simulink model "OSWEC"  (R2025b)
settings: Solver=ode14x  StartTime=0  StopTime=400  FixedStep=0.01  MaxStep=0.01  RelTol=1e-3  EnableMultiTasking=on
values from neighbouring files (symbols this model uses):
  accVolHP = 50*0.5    (= 25)    [VariableDefinition.m]
  crankLength = 3    [VariableDefinition.m]
  Dmax = 42    [VariableDefinition.m]
  genShaftSpeedRef = 1800    [VariableDefinition.m]
  iGainGen = 1    [VariableDefinition.m]
  m3persecond2lpm = 1000*60    (= 60000)    [VariableDefinition.m]
  offsetLength = 1.3    [VariableDefinition.m]
  pa2psi = 1/6894.75    (= 0.000145037891149)    [VariableDefinition.m]
  pGainGen = 5    [VariableDefinition.m]
  radsec2rpm = 60/(2*pi)    (= 9.54929658551)    [VariableDefinition.m]
  rodLength = 5    [VariableDefinition.m]
undefined symbols (not defined in the file or in its folder): body, constraint, pto
libraries: fl_lib x55, nesl_utility x28, sh_lib x9, WECSim_Lib_Body_Elements x2, WECSim_Lib_Constraints x1, WECSim_Lib_Frames x1, WECSim_Lib_PTOs x1, slpidlib x1, sdl_lib x1
settings Model: Creator=mlawson  LastModifiedBy=jleonqu
settings SolverCC: ZeroCrossControl=DisableAll  AlgebraicLoopSolver=LineSearch  AutoInsertRateTranBlk=on
settings DataIOCC: SaveFormat=Array  SaveOutput=off  SaveTime=off  ReturnWorkspaceOutputs=off
settings OptimizationCC: LifeSpan=inf  SimCompilerOptimization=on
settings DebuggingCC: MergeDetectMultiDrivingBlocksExec=none  SolverPrmCheckMsg=warning  UnconnectedInputMsg=warning  UnconnectedOutputMsg=warning  UnconnectedLineMsg=warning  AllowSymbolicDim=off  StateNameClashWarn=warning  SFUnexpectedBacktrackingDiag=warning  SFNoUnconditionalDefaultTransitionDiag=warning  SFExecutionAtInitializationDiag=none  ArithmeticOperatorsInVariantConditions=warning
settings HardwareCC: ProdBitPerPointer=32.0  ProdBitPerSizeT=32.0  ProdBitPerPtrDiffT=32.0  ProdLargestAtomicFloat=None  ProdIntDivRoundTo=Undefined  ProdEndianess=Unspecified  ProdWordSize=32.0  ProdHWDeviceType=32-bit Generic
settings ModelReferenceCC: EnableRefExpFcnMdlSchedulingChecks=on  PropagateSignalLabelsOutOfModel=off
settings SFSimCC: SimUseLocalCustomCode=off  CustomCodeUndefinedFunction=UseInterfaceOnly
settings RTWCC: RTWUseLocalCustomCode=off  GPUComputeCapability=3.5  DLArmComputeVersion=19.05
settings CodeAppCC: StateflowObjectComments=on
settings GRTTargetCC: TargetLangStandard=C89/C90 (ANSI)
settings ConfigComp: CovMetricSettings=dw  CovSaveCumulativeToWorkspaceVar=on  CovSaveSingleToWorkspaceVar=on  CovExternalEMLEnable=off  CovSFcnEnable=off
settings SimscapeCC: SimscapeNormalizeSystem=off
settings ConfigurationSet: Description=SimMechanics 2G
settings ExplorerConfigSet: SimMechanicsOpenEditorOnUpdate=off  InternalSimMechanicsExplorerSettings="<ExplorerConfiguration><canonicalview>default</canonicalview><TilePanel><TileInfo><Tiles Columns=\"1\" Count=\"1\" Rows=\"1\"><Column Left=\"2\" Weight=\"1\"/><Column Left=\"1335\"/><Row Top=\"2\" Weight=\"1\"/><Row Top=\"911\"/><Tile Height=\"1\" Width=\"1\" X=\"0\" Y=\"0\"/></Tiles></TileInfo><SceneInfo><SceneViewer><BGColor><R>0.60000002384185791</R><G>0.60000002384185791</G><B>0.60000002384185791</B></BGColor><Camera><Position><X>365.37645888990272</X><Y>-369.82486814446582</Y><Z>359.64809521743916</Z></Position><Center><X>-6.7351450971904585</X><Y>2.2867358426280204</Y><Z>-12.463508769654169</Z></Center><Up><X>-0.40824829046386307</X><Y>0.40824829046386307</Y><Z>0.81649658092772615</Z></Up><Left>-57.820127362122818</Left><Right>57.820127362122818</Right><Bottom>-38.308817187253304</Bottom><Top>38.308817187253304</Top></Camera></SceneViewer></SceneInfo></TilePanel></ExplorerConfiguration>"

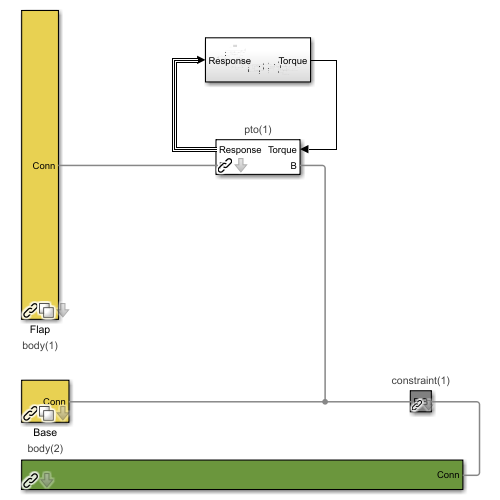
[thumbnail: Simulink's stored preview of the top-level diagram]
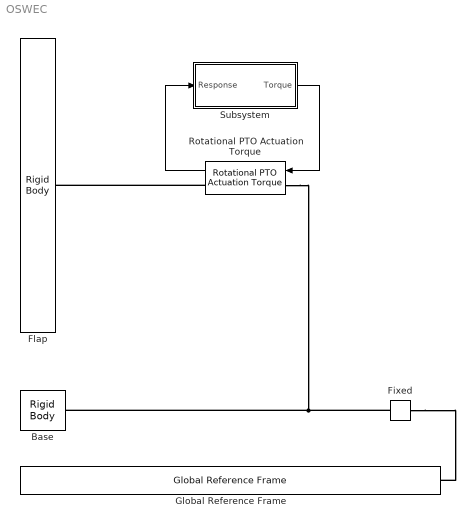
== system OSWEC ==
  Base : WECSim_Lib_Body_Elements/Rigid Body  body=body(2)
      settings: SourceProductName=WEC-Sim
  Fixed : WECSim_Lib_Constraints/Fixed  constraint=constraint(1)
      settings: AttributesFormatString=%<constraint>  SourceProductName=WEC-Sim
  Flap : WECSim_Lib_Body_Elements/Rigid Body  body=body(1)
      settings: SourceProductName=WEC-Sim
  Global Reference Frame : WECSim_Lib_Frames/Global Reference Frame  waves=waves  simu=simu
      settings: SourceProductName=WEC-Sim
  Rotational PTO Actuation Torque : WECSim_Lib_PTOs/Rotational PTO Actuation Torque  pto=pto(1)
      settings: AttributesFormatString=%<pto>
  Subsystem : Subsystem
  wires:
  Rotational PTO Actuation Torque/1 -> Subsystem/1(Response)
  Subsystem/1(Torque) -> Rotational PTO Actuation Torque/1
  connections:
  Fixed/LConn1 -- Global Reference Frame/RConn1
  Fixed/RConn1 -- Rotational PTO Actuation Torque/LConn1 -- Base/RConn1
  Rotational PTO Actuation Torque/RConn1 -- Flap/RConn1

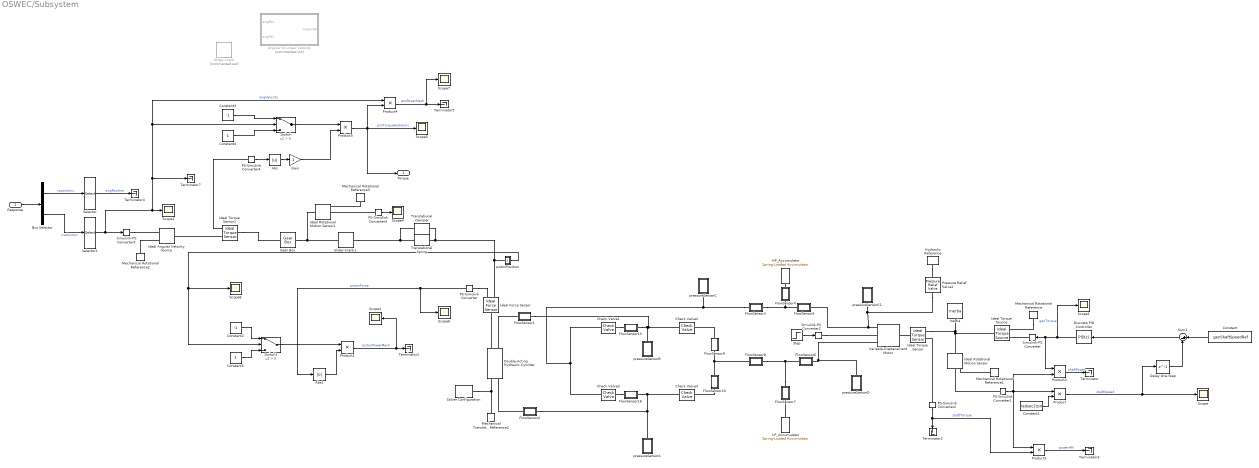
== system OSWEC/Subsystem ==
  Response : Inport
  Abs : Abs  SaturateOnIntegerOverflow=off
  Abs1 : Abs  SaturateOnIntegerOverflow=off
  Angular to Linear Velocity : Subsystem  Commented=on  AncestorBlock=|
      | WECSim_Lib_PTOSim/Motion Conversion/Rotary to Linear
      | Crank/Angular to Linear
      | Velocity
  Bus Selector : BusSelector  OutputSignals=position,velocity
  Check Valve1 : sh_lib/Valves/Directional Valves/Check Valve  area_max=areaMaxValve m^2  pres_crack=pCrack psi  pres_max=pMaxValve psi  C_d=0.7  A_leak=1e-12 m^2  lam_spec=1  B_lam=0.999  Re_cr=12  dynamic=0  tau=0.1 s  area_init=1e-12 m^2
      settings: InternalSimscapePortConfiguration="{\"Bottom\":[],\"Left\":[{\"id\":\"A\",\"label\":\"A\",\"type\":\"foundation.hydraulic.hydraulic\"}],\"Right\":[{\"id\":\"B\",\"label\":\"B\",\"type\":\"foundation.hydraulic.hydraulic\"}],\"Top\":[]}"
  Check Valve2 : sh_lib/Valves/Directional Valves/Check Valve  area_max=areaMaxValveLP m^2  pres_crack=pCrackLP psi  pres_max=pMaxValveLP psi  C_d=0.7  A_leak=1e-12 m^2  lam_spec=1  B_lam=0.999  Re_cr=12  dynamic=0  tau=0.1 s  area_init=1e-12 m^2
      settings: InternalSimscapePortConfiguration="{\"Bottom\":[],\"Left\":[{\"id\":\"A\",\"label\":\"A\",\"type\":\"foundation.hydraulic.hydraulic\"}],\"Right\":[{\"id\":\"B\",\"label\":\"B\",\"type\":\"foundation.hydraulic.hydraulic\"}],\"Top\":[]}"
  Check Valve3 : sh_lib/Valves/Directional Valves/Check Valve  area_max=areaMaxValve m^2  pres_crack=pCrack psi  pres_max=pMaxValve psi  C_d=0.7  A_leak=1e-12 m^2  lam_spec=1  B_lam=0.999  Re_cr=12  dynamic=0  tau=0.1 s  area_init=1e-12 m^2
      settings: InternalSimscapePortConfiguration="{\"Bottom\":[],\"Left\":[{\"id\":\"A\",\"label\":\"A\",\"type\":\"foundation.hydraulic.hydraulic\"}],\"Right\":[{\"id\":\"B\",\"label\":\"B\",\"type\":\"foundation.hydraulic.hydraulic\"}],\"Top\":[]}"
  Check Valve4 : sh_lib/Valves/Directional Valves/Check Valve  area_max=areaMaxValveLP m^2  pres_crack=pCrackLP psi  pres_max=pMaxValveLP psi  C_d=0.7  A_leak=1e-12 m^2  lam_spec=1  B_lam=0.999  Re_cr=12  dynamic=0  tau=0.1 s  area_init=1e-12 m^2
      settings: InternalSimscapePortConfiguration="{\"Bottom\":[],\"Left\":[{\"id\":\"A\",\"label\":\"A\",\"type\":\"foundation.hydraulic.hydraulic\"}],\"Right\":[{\"id\":\"B\",\"label\":\"B\",\"type\":\"foundation.hydraulic.hydraulic\"}],\"Top\":[]}"
  Constant : Constant  Value=genShaftSpeedRef
  Constant1 : Constant  Value=radsec2rpm
  Constant2 : Constant  Value=-1
  Constant3 : Constant  Value=-1
  Constant4 : Constant
  Constant5 : Constant
  Delay One Step : Delay  DelayLength=1
  Discrete PID Controller : slpidlib/PID Controller  Controller=PID  Form=Parallel  TimeDomain=Discrete-time  UseExternalTs=off  SampleTime=-1  IntegratorMethod=Forward Euler  FilterMethod=Forward Euler  ControllerParametersSource=internal  P=pGainGen  I=iGainGen  UseKiTs=off  D=0  UseExternalDerivativeSource=off  N=100  UseFilter=off  TunerSelectOption=Transfer Function Based (PID Tuner App)  InitialConditionSource=internal  InitialConditionForIntegrator=0  InitialConditionForFilter=0  DifferentiatorICPrevScaledInput=0  ExternalReset=none  TrackingMode=off  Kt=1  LimitOutput=off  SatLimitsSource=internal  UpperSaturationLimit=inf  LowerSaturationLimit=-inf  LinearizeAsGain=off  AntiWindupMode=none  Kb=1  LimitIntegrator=off  UpperIntegratorSaturationLimit=inf  LowerIntegratorSaturationLimit=-inf  POutMin=[]  POutMax=[]  IOutMin=[]  IOutMax=[]  DOutMin=[]  DOutMax=[]  NOutMin=[]  NOutMax=[]  SumOutMin=[]  SumOutMax=[]  SaturationOutMin=[]  SaturationOutMax=[]  PParamMin=[]  PParamMax=[]  IParamMin=[]  IParamMax=[]  DParamMin=[]  DParamMax=[]  NParamMin=[]  NParamMax=[]  KbParamMin=[]  KbParamMax=[]  KtParamMin=[]  KtParamMax=[]  KbOutMin=[]  KbOutMax=[]  KtOutMin=[]  KtOutMax=[]  IntegratorOutMin=[]  IntegratorOutMax=[]  FilterOutMin=[]  FilterOutMax=[]  SumI1OutMin=[]  SumI1OutMax=[]  SumI2OutMin=[]  SumI2OutMax=[]  SumI3OutMin=[]  SumI3OutMax=[]  SumI4OutMin=[]  SumI4OutMax=[]  SumDOutMin=[]  SumDOutMax=[]  DifferentiatorOutMin=[]  DifferentiatorOutMax=[]  FilterDiffOutCoefMin=[]  FilterDiffOutCoefMax=[]  ReciprocalOutMin=[]  ReciprocalOutMax=[]  SumDenOutMin=[]  SumDenOutMax=[]  SumNumOutMin=[]  SumNumOutMax=[]  DivideOutMin=[]  DivideOutMax=[]  UdiffTsProdOutMin=[]  UdiffTsProdOutMax=[]  NTsProdOutMin=[]  NTsProdOutMax=[]  UintegralTsProdOutMin=[]  UintegralTsProdOutMax=[]  UngainTsProdOutMin=[]  UngainTsProdOutMax=[]  ClampingZeroOutDataTypeStr=Inherit: Inherit via back propagation  ClampingZeroOutMin=[]  ClampingZeroOutMax=[]  FilterDenConstantOutDataTypeStr=Inherit: Inherit via back propagation  FilterDenConstantOutMin=[]  FilterDenConstantOutMax=[]  PCopyOutDataTypeStr=Inherit: Inherit via back propagation  PCopyOutMin=[]  PCopyOutMax=[]  NCopyOutDataTypeStr=Inherit: Inherit via back propagation  NCopyOutMin=[]  NCopyOutMax=[]  IntegratorContinuousStateAttributes=''  IntegratorStateMustResolveToSignalObject=off  IntegratorRTWStateStorageClass=Auto  FilterContinuousStateAttributes=''  FilterStateMustResolveToSignalObject=off  FilterRTWStateStorageClass=Auto  ParallelPVariant=InternalParameters  IdealPVariant=Disabled  IVariant=InternalParameters  DVariant=InternalParameters  IntegratorVariant=Discrete  SatVariant=Disabled  AWVariant=Passthrough  PCopyVariant=Disabled  TRVariant=Disabled  FdbkBlocksVariant=Forward  IdealPFdbkVariant=Disabled  SatFdbkVariant=Disabled  DerivativeFilterVariant=Differentiator  NVariant=Passthrough  NCopyVariant=Disabled_SignalSpec  FilterICVariant=InternalICsDifferentiator  IntegratorICVariant=InternalICs  ExternalResetVariant=Disabled  TRSumVariant=Passthrough  SumFdbkVariant=Disabled  SumVariant=Sum_PID  TsampFilterVariant=InternalTs  TsampNgainVariant=Passthrough  TsampIntegralVariant=Disabled_SignalSpec  ExternalSaturationOutDataTypeStr=Inherit: Same as second input  DerivativeSourceVariant=ErrorSignal  PreIntVariant=InternalPreInt
      settings: LibrarySourceBlock=simulink/Discrete/Discrete PID Controller
  Double-Acting Hydraulic Cylinder : sh_lib/Hydraulic Cylinders/Double-Acting Hydraulic Cylinder  area_A=areaHC m^2  area_B=areaHC m^2  stroke=strokePiston m  dead_vol_A=deadVolume m^3  dead_vol_B=deadVolume m^3  k_sh=1.4  or=sh.cylinders.enum.MechOrientationTranslational.Positive  stiff=1e6 N/m  D=150 N*s/m  hardstop_model=1  transition=0.1 mm  displacement_spec=foundation.enum.DisplacementSpec.Calculate  init_pos=pistonInitialPos m  init_pressure_A=0 Pa  init_pressure_B=0 Pa
      settings: InternalSimscapePortConfiguration="{\"Bottom\":[],\"Left\":[{\"id\":\"C\",\"label\":\"C\",\"type\":\"foundation.mechanical.translational.translational\"},{\"id\":\"A\",\"label\":\"A\",\"type\":\"foundation.hydraulic.hydraulic\"}],\"Right\":[{\"id\":\"R\",\"label\":\"R\",\"type\":\"foundation.mechanical.translational.translational\"},{\"id\":\"B\",\"label\":\"B\",\"type\":\"foundation.hydraulic.hydraulic\"}],\"Top\":[]}"
  FlowSensor1 : Subsystem
  FlowSensor10 : Subsystem
  FlowSensor13 : Subsystem
  FlowSensor16 : Subsystem
  FlowSensor2 : Subsystem
  FlowSensor3 : Subsystem
  FlowSensor4 : Subsystem
  FlowSensor5 : Subsystem
  FlowSensor6 : Subsystem
  FlowSensor7 : Subsystem
  FlowSensor8 : Subsystem
  FlowSensor9 : Subsystem
  Gain : Gain
  Gear Box : fl_lib/Mechanical/Mechanisms/Gear Box  ratio=1/5  t_in_specify=off  t_in_priority=None  t_in=0 N*m  t_in_nominal_specify=off  t_in_nominal_value=1  t_in_nominal_unit=N*m  t_out_specify=off  t_out_priority=None  t_out=0 N*m  t_out_nominal_specify=off  t_out_nominal_value=1  t_out_nominal_unit=N*m
  HP_Accumulator : sh_lib/Accumulators/Spring-Loaded Accumulator  capacity=accVolHP l  pr_preload=pPreLoadHP psi  pr_max=pMaxAccHP psi  stiff_coeff=1e10 Pa/m^3  penetr_coeff=1e10 Pa*s/m^6  flow_rate_specify=off  flow_rate_priority=None  flow_rate=5e-3 m^3/s  flow_rate_nominal_specify=off  flow_rate_nominal_value=1  flow_rate_nominal_unit=m^3/s  fluid_volume_specify=off  fluid_volume_priority=High  fluid_volume=accVolHP*0.01 l  fluid_volume_nominal_specify=off  fluid_volume_nominal_value=1  fluid_volume_nominal_unit=m^3  fluid_pressure_specify=off  fluid_pressure_priority=None  fluid_pressure=1.01325e5 Pa  fluid_pressure_nominal_specify=off  fluid_pressure_nominal_value=1  fluid_pressure_nominal_unit=Pa
      settings: InternalSimscapePortConfiguration="{\"Bottom\":[],\"Left\":[],\"Right\":[{\"id\":\"A\",\"label\":\"A\",\"type\":\"foundation.hydraulic.hydraulic\"}],\"Top\":[]}"
  Hydraulic Reference : fl_lib/Hydraulic/Hydraulic Elements/Hydraulic Reference
  Ideal Angular Velocity Source : fl_lib/Mechanical/Mechanical Sources/Ideal Angular Velocity Source
  Ideal Force Sensor : fl_lib/Mechanical/Mechanical Sensors/Ideal Force Sensor
  Ideal Rotational Motion Sensor : fl_lib/Mechanical/Mechanical Sensors/Ideal Rotational Motion Sensor  reference=foundation.enum.MeasurementReference.difference  acceleration_port=false  velocity_port=true  position_port=true  wrap_angle=false  offset=0 rad
  Ideal Rotational Motion Sensor1 : fl_lib/Mechanical/Mechanical Sensors/Ideal Rotational Motion Sensor  reference=foundation.enum.MeasurementReference.difference  acceleration_port=false  velocity_port=true  position_port=true  wrap_angle=false  offset=0 rad
  Ideal Torque Sensor : fl_lib/Mechanical/Mechanical Sensors/Ideal Torque Sensor
  Ideal Torque Sensor1 : fl_lib/Mechanical/Mechanical Sensors/Ideal Torque Sensor
  Ideal Torque Source : fl_lib/Mechanical/Mechanical Sources/Ideal Torque Source
  Inertia : fl_lib/Mechanical/Rotational Elements/Inertia  inertia=50 kg*m^2  num_ports=foundation.enum.numPorts2.one  w_specify=off  w_priority=High  w=genShaftSpeedRef rpm  w_nominal_specify=off  w_nominal_value=1  w_nominal_unit=rad/s  t_specify=off  t_priority=None  t=0 N*m  t_nominal_specify=off  t_nominal_value=1  t_nominal_unit=N*m
  LP_Accumulator : sh_lib/Accumulators/Spring-Loaded Accumulator  capacity=accVolLP l  pr_preload=pPreLoadLP psi  pr_max=pMaxAccLP psi  stiff_coeff=1e10 Pa/m^3  penetr_coeff=1e10 Pa*s/m^6  flow_rate_specify=off  flow_rate_priority=None  flow_rate=5e-3 m^3/s  flow_rate_nominal_specify=off  flow_rate_nominal_value=1  flow_rate_nominal_unit=m^3/s  fluid_volume_specify=off  fluid_volume_priority=High  fluid_volume=accVolLP m^3  fluid_volume_nominal_specify=off  fluid_volume_nominal_value=1  fluid_volume_nominal_unit=m^3  fluid_pressure_specify=off  fluid_pressure_priority=None  fluid_pressure=1.01325e5 Pa  fluid_pressure_nominal_specify=off  fluid_pressure_nominal_value=1  fluid_pressure_nominal_unit=Pa
      settings: InternalSimscapePortConfiguration="{\"Bottom\":[],\"Left\":[],\"Right\":[{\"id\":\"A\",\"label\":\"A\",\"type\":\"foundation.hydraulic.hydraulic\"}],\"Top\":[]}"
  Mechanical Rotational Reference{,1..3} (4 alike) : fl_lib/Mechanical/Rotational Elements/Mechanical Rotational Reference
  Mechanical Translational Reference2 : fl_lib/Mechanical/Translational Elements/Mechanical Translational Reference
  PS-Simulink Converter{,1..4} (5 alike) : nesl_utility/PS-Simulink Converter  PhysicalDomain=network_engine_domain  SubClassName=ps_output  LeftPortType=input  RightPortType=output  PseudoPeriodic=off  Frequencies=[]  VectorFormat=inherit  Unit=inherit  AffineConversion=off
  Pressure Relief Valve2 : sh_lib/Valves/Pressure Control Valves/Pressure Relief Valve  valve_area_spec=1  p_diff_TLU=[30.15e5 : 15e3 : 31.35e5] Pa  area_TLU=[1 : 1 : 9] .* 1e-5 m^2  area_max=2.2e-4 m^2  pres_set=4900 psi  reg_range=10 psi  C_d=0.7  A_leak=1e-12 m^2  lam_spec=1  B_lam=0.999  Re_cr=12  dynamic=0  tau=0.1 s  area_init=1e-12 m^2
      settings: InternalSimscapePortConfiguration="{\"Bottom\":[],\"Left\":[{\"id\":\"A\",\"label\":\"A\",\"type\":\"foundation.hydraulic.hydraulic\"}],\"Right\":[{\"id\":\"B\",\"label\":\"B\",\"type\":\"foundation.hydraulic.hydraulic\"}],\"Top\":[]}"
  Product{,1..5} (6 alike) : Product
  Scope{,1..8} (9 alike) : Scope
      Scope settings: ActiveDisplayYMinimum=1738.7756957222209  ActiveDisplayYMaximum=1946.7249509603892
      Scope1 settings: ActiveDisplayYMinimum=-94.135566599802871  ActiveDisplayYMaximum=67.441074091156352
      Scope2 settings: ActiveDisplayYMinimum=-0.31429832837768534  ActiveDisplayYMaximum=0.30729177387363948  DataLoggingVariableName=ScopeData2
      Scope3 settings: ActiveDisplayYMinimum=-0.10262196705005888  ActiveDisplayYMaximum=0.14966467708972742  DataLoggingVariableName=ScopeData8
      Scope4 settings: ActiveDisplayYMinimum=-3.77179135660224  ActiveDisplayYMaximum=3.7759988528286708  DataLoggingVariableName=ScopeData9
      Scope5 settings: ActiveDisplayYMinimum=-1.4215512241951279E+7  ActiveDisplayYMaximum=1.4218962302598771E+7  DataLoggingVariableName=ScopeData10
      Scope6 settings: ActiveDisplayYMinimum=-1.9695787856257146E+6  ActiveDisplayYMaximum=1.571747168448562E+6  DataLoggingVariableName=ScopeData11
      Scope7 settings: ActiveDisplayYMinimum=-1.8232047357809118E+6  ActiveDisplayYMaximum=202578.3039756568  DataLoggingVariableName=ScopeData12
      Scope8 settings: DataLoggingVariableName=ScopeData13
  Selector : Selector  InputPortWidth=6  IndexOptions=Index vector (dialog)  Indices=5  OutputSizes=1
  Selector1 : Selector  InputPortWidth=6  IndexOptions=Index vector (dialog)  Indices=5  OutputSizes=1
  Simulink-PS Converter : nesl_utility/Simulink-PS Converter  PhysicalDomain=network_engine_domain  SubClassName=ps_input  LeftPortType=input  RightPortType=output  PseudoPeriodic=off  Frequencies=[]  NoiseDistribution=none  NoiseParameters=[]  Unit=1  AffineConversion=off  FilteringAndDerivatives=provide  SimscapeFilterOrder=1  InputFilterTimeConstant=0.001  UdotUserProvided=0
  Simulink-PS Converter2 : nesl_utility/Simulink-PS Converter  PhysicalDomain=network_engine_domain  SubClassName=ps_input  LeftPortType=input  RightPortType=output  PseudoPeriodic=off  Frequencies=[]  NoiseDistribution=none  NoiseParameters=[]  Unit=1  AffineConversion=off  FilteringAndDerivatives=provide  SimscapeFilterOrder=1  InputFilterTimeConstant=0.001  UdotUserProvided=0
  Simulink-PS Converter3 : nesl_utility/Simulink-PS Converter  PhysicalDomain=network_engine_domain  SubClassName=ps_input  LeftPortType=input  RightPortType=output  PseudoPeriodic=off  Frequencies=[]  NoiseDistribution=none  NoiseParameters=[]  Unit=1  AffineConversion=off  FilteringAndDerivatives=filter  SimscapeFilterOrder=1  InputFilterTimeConstant=0.001  UdotUserProvided=0
  Slider-Crank : fl_lib/Mechanical/Mechanisms/Slider-Crank  Commented=on  crank=crankLength m  rod=rodLength m  inertia=0.01 kg*m^2  k=1e6 N/m  b=1e3 N*s/m  theta_specify=off  theta_priority=High  theta=pi / 2 rad  theta_nominal_specify=off  theta_nominal_value=1  theta_nominal_unit=rad  w_specify=off  w_priority=High  w=0 rad/s  w_nominal_specify=off  w_nominal_value=1  w_nominal_unit=rad/s
      settings: InternalSimscapePortConfiguration="{\"Bottom\":[],\"Left\":[{\"id\":\"C\",\"label\":\"C\",\"type\":\"foundation.mechanical.rotational.rotational\"}],\"Right\":[{\"id\":\"S\",\"label\":\"S\",\"type\":\"foundation.mechanical.translational.translational\"}],\"Top\":[]}"
  Slider-Crank1 : fl_lib/Mechanical/Mechanisms/Slider-Crank  crank=2 m  rod=4 m  inertia=0.01 kg*m^2  k=1e6 N/m  b=1e3 N*s/m  theta_specify=off  theta_priority=High  theta=pi / 2 rad  theta_nominal_specify=off  theta_nominal_value=1  theta_nominal_unit=rad  w_specify=off  w_priority=High  w=0 rad/s  w_nominal_specify=off  w_nominal_value=1  w_nominal_unit=rad/s
      settings: InternalSimscapePortConfiguration="{\"Bottom\":[],\"Left\":[{\"id\":\"C\",\"label\":\"C\",\"type\":\"foundation.mechanical.rotational.rotational\"}],\"Right\":[{\"id\":\"S\",\"label\":\"S\",\"type\":\"foundation.mechanical.translational.translational\"}],\"Top\":[]}"
  Solver Configuration : nesl_utility/Solver Configuration  PhysicalDomain=network_engine_domain  SubClassName=solver  LeftPortType=input  RightPortType=generic  Tones=[]  Harmonics=[]  SimulateNoise=off  Profile=off  UseLocalSampling=off  EnableSwitchedLinearOptims=on  FrequencyDomain=off  UseCCode=off  RelTol=0.001  AbsTol=0.001  MinStep=1e-09  ToWorkspace=off  RevertToSquareIcSolve=off  NumHomotopyIterations=100  PhasorMode=off  PhasorModeNumHarmonics=1  ConsistencySolver=NEWTON_XTOL_AFTER_FTOL  IndexReductionMethod=DerivativeReplacement  DoDC=off  ResidualTolerance=1e-09  ConsistencyTolSource=GLOBAL  ConsistencyAbsTol=0.001  ConsistencyRelTol=0.001  ConsistencyTolFactor=0.001  UseLocalSolver=off  LocalSolverChoice=NE_BACKWARD_EULER_ADVANCER  ResolveIndetEquations=on  FunctionEvalNumThread=1  LocalSolverSampleTime=0.001  DoFixedCost=off  MaxNonlinIter=3  MaxModeIter=2  ComputeImpulses=off  ImpulseIterations=2  LinearAlgebra=auto  LinearAlgebraNumThread=0  EquationFormulation=NE_TIME_EF  DelaysMemoryBudget=1024  AutomaticFiltering=on  FilteringTimeConstant=0.001  PartitionStorageMethod=AS_NEEDED  PartitionMemoryBudget=1024  PartitionMethod=ROBUST  MultibodyUseLocalSolver=off  MultibodyLocalSolverChoice=ODE1  MultibodyLocalSolverSampleTime=0.001
  Step : Step  Time=100  Before=0.0075  After=0.0075  SampleTime=0
  Sum1 : Sum  Inputs=|+-
  Switch : Switch  Criteria=u2 > Threshold  SaturateOnIntegerOverflow=off  InputSameDT=off
  Switch1 : Switch  Criteria=u2 > Threshold  SaturateOnIntegerOverflow=off  InputSameDT=off
  Terminator{,1..5,7} (7 alike) : Terminator
  Translational Damper : sdl_lib/Couplings & Drives/Springs & Dampers/Translational Damper  D=14000 N*s/m  thermal_port=simscape.enum.thermaleffects.omit  thermal_mass=50 kJ/K  temperature_specify=off  temperature_priority=High  temperature=300 K  temperature_nominal_specify=off  temperature_nominal_value=1  temperature_nominal_unit=K
  Translational Spring : fl_lib/Mechanical/Translational Elements/Translational Spring  spr_rate=1e7 N/m  v_specify=off  v_priority=None  v=0 m/s  v_nominal_specify=off  v_nominal_value=1  v_nominal_unit=m/s  f_specify=off  f_priority=None  f=0 N  f_nominal_specify=off  f_nominal_value=1  f_nominal_unit=N  x_specify=off  x_priority=High  x=0 m  x_nominal_specify=off  x_nominal_value=1  x_nominal_unit=m
  Variable-Displacement Motor : sh_lib/Pumps and Motors/Variable-Displacement Motor  mdl_type=2  stroke_max=0.005 m  D_max=Dmax cm^3/rev  cntrl_mem_tab="[-.0075, 0,  .0075] m"  displ_tab=[-Dmax, 0, Dmax] cm^3/rev  interp_method=1  extrap_method=1  loss_spec=1  w_nominal=shaftSpeedNominal rpm  pr_nominal=pressureNom psi  visc_nominal=kinematicVisNom cSt  dens_nominal=fluidDensityNom kg/m^3  efficiency_vol=0.92  no_load_torque=noLoadTorque N*m  torque_pressure_coeff=frictionTorqueVsPressure N*m/Pa  p_diff_eff_TLU=[100000, 1000000, 2000000] Pa  omega_eff_TLU=[25, 50, 100, 200, 300, 400] rad/s  displacement_eff_TLU=[-30, -19, 19, 30] cm^3/rev  vol_eff_TLU=repmat([.816, .908, .954, .977, .981, .984; .325, .663, .831, .916, .925, .946; .137, .568, .78, .892, .893, .91], 1, 1, 4)  mech_eff_TLU=repmat([.996, .996, .996, .996, .996, .996; .988, .989, .989, .989, .989, .99; .981, .981, .982, .982, .983, .984], 1, 1, 4)  p_diff_loss_TLU=[100000, 1000000, 2000000] Pa  omega_loss_TLU=[25, 50, 100, 200, 300, 400] rad/s  displacement_loss_TLU=[-30, -19, 19, 30] cm^3/rev  vol_loss_TLU=repmat([.0282, .0253, .0241, .0235, .0291, .0325; .2596, .1271, .1017, .0917, .1216, .1142; .7874, .1901, .141, .1211, .1797, .1978] * 1e-3, 1, 1, 4) m^3/s  mech_loss_TLU=repmat([.002, .002, .002, .002, .002, .002; .06, .055, .055, .055, .055, .05; .19, .19, .18, .18, .17, .16], 1, 1, 4) N*m  pressure_threshold=1e5 Pa  omega_threshold=10 rad/s  displacement_threshold=0.5 cm^3/rev  octant_check=0  pressure_check=0  min_valid_pressure=0 Pa  vol_eff_min=1e-3  vol_eff_max=1  mech_eff_min=1e-3  mech_eff_max=1
      settings: InternalSimscapePortConfiguration="{\"Bottom\":[],\"Left\":[{\"id\":\"A\",\"label\":\"A\",\"type\":\"foundation.hydraulic.hydraulic\"},{\"id\":\"C\",\"label\":\"C\",\"type\":\"input\"},{\"id\":\"B\",\"label\":\"B\",\"type\":\"foundation.hydraulic.hydraulic\"}],\"Right\":[{\"id\":\"S\",\"label\":\"S\",\"type\":\"foundation.mechanical.rotational.rotational\"}],\"Top\":[]}"
  pistonPosition : Subsystem
  pressureSensorA : Subsystem
  pressureSensorB : Subsystem
  pressureSensorC : Subsystem
  pressureSensorC1 : Subsystem
  pressureSensorD : Subsystem
  Torque : Outport
  wires:
  PS-Simulink Converter2/1 -> Product3/2, Terminator2/1  "shaftTorque"
  Constant/1 -> Sum1/1
  PS-Simulink Converter1/1 -> Product2/2, Product3/1, Product/1
  Sum1/1 -> Discrete PID Controller/1
  Product1/1 -> Scope3/1, Terminator1/1  "pistonPowerMech"
  Product2/1 -> Terminator/1  "shaftPower"
  Product3/1 -> Terminator3/1  "powerHM"
  PS-Simulink Converter/1 -> Scope6/1, Abs1/1  "pistonForce"
  Step/1 -> Simulink-PS Converter2/1
  Discrete PID Controller/1 -> Product2/1, Simulink-PS Converter/1, Scope1/1  "genTorque"
  Product/1 -> Delay One Step/1, Scope/1  "shaftSpeed"
  Constant1/1 -> Product/2
  Response/1 -> Bus Selector/1
  Bus Selector/1 -> Selector/1  "<position>"
  Selector/1 -> Terminator4/1  "angPosition"
  Bus Selector/2 -> Selector1/1  "<velocity>"
  Selector1/1 -> Product4/1, Switch/2, Terminator7/1, Scope2/1, Simulink-PS Converter3/1  "angVelocity"
  Delay One Step/1 -> Sum1/2
  PS-Simulink Converter3/1 -> Scope4/1
  PS-Simulink Converter4/1 -> Abs/1
  Product4/1 -> Scope7/1, Terminator5/1  "ptoPowerMech"
  Abs/1 -> Gain/1
  Constant3/1 -> Switch/1
  Constant4/1 -> Switch/3
  Switch/1 -> Product5/1
  Gain/1 -> Product5/2
  Product5/1 -> Torque/1, Product4/2, Scope5/1  "ptoTorqueHydraulic"
  Switch1/1 -> Product1/1
  pistonPosition/1(Out1) -> Switch1/2, Scope8/1
  Constant2/1 -> Switch1/1
  Constant5/1 -> Switch1/3
  Abs1/1 -> Product1/2
  connections:
  Check Valve4/RConn1 -- FlowSensor16/LConn1 -- FlowSensor2/RConn1 -- pressureSensorA/LConn1
  FlowSensor9/LConn1 -- FlowSensor8/RConn1 -- FlowSensor10/LConn1
  FlowSensor13/LConn1 -- FlowSensor1/RConn1 -- Check Valve2/RConn1 -- pressureSensorB/LConn1
  pressureSensorC1/LConn1 -- Variable-Displacement Motor/LConn1 -- FlowSensor5/RConn1 -- Pressure Relief Valve2/LConn1
  FlowSensor4/LConn1 -- FlowSensor5/LConn1 -- FlowSensor3/RConn1
  Inertia/LConn1 -- Ideal Rotational Motion Sensor/LConn1 -- Ideal Torque Source/LConn1 -- Ideal Torque Sensor/RConn1
  pressureSensorD/LConn1 -- FlowSensor6/LConn1 -- Variable-Displacement Motor/LConn3
  pistonPosition/LConn1 -- Translational Damper/RConn1 -- Translational Spring/RConn1 -- Ideal Force Sensor/RConn1
  FlowSensor7/LConn1 -- FlowSensor6/RConn1 -- FlowSensor8/LConn1
  FlowSensor3/LConn1 -- Check Valve3/RConn1 -- Check Valve1/RConn1 -- pressureSensorC/LConn1
  Solver Configuration/RConn1 -- Mechanical Translational Reference2/LConn1 -- Double-Acting Hydraulic Cylinder/LConn1
  FlowSensor10/RConn1 -- Check Valve4/LConn1
  FlowSensor9/RConn1 -- Check Valve2/LConn1
  Check Valve1/LConn1 -- FlowSensor13/RConn1
  Hydraulic Reference/LConn1 -- Pressure Relief Valve2/RConn1
  PS-Simulink Converter/LConn1 -- Ideal Force Sensor/RConn2
  Simulink-PS Converter/RConn1 -- Ideal Torque Source/RConn1
  Mechanical Rotational Reference1/LConn1 -- Ideal Rotational Motion Sensor/RConn1
  FlowSensor2/LConn1 -- Double-Acting Hydraulic Cylinder/LConn2
  Simulink-PS Converter2/RConn1 -- Variable-Displacement Motor/LConn2
  FlowSensor1/LConn1 -- Double-Acting Hydraulic Cylinder/RConn2
  FlowSensor4/RConn1 -- HP_Accumulator/RConn1
  Ideal Torque Sensor/LConn1 -- Variable-Displacement Motor/RConn1
  PS-Simulink Converter1/LConn1 -- Ideal Rotational Motion Sensor/RConn2
  LP_Accumulator/RConn1 -- FlowSensor7/RConn1
  Ideal Force Sensor/LConn1 -- Double-Acting Hydraulic Cylinder/RConn1
  PS-Simulink Converter2/LConn1 -- Ideal Torque Sensor/RConn2
  Mechanical Rotational Reference/LConn1 -- Ideal Torque Source/RConn2
  Check Valve3/LConn1 -- FlowSensor16/RConn1
  Simulink-PS Converter3/RConn1 -- Ideal Angular Velocity Source/RConn1
  Gear Box/RConn1 -- Ideal Rotational Motion Sensor1/LConn1 -- Slider-Crank1/LConn1
  Mechanical Rotational Reference2/LConn1 -- Ideal Angular Velocity Source/RConn2
  Mechanical Rotational Reference3/LConn1 -- Ideal Rotational Motion Sensor1/RConn1
  PS-Simulink Converter3/LConn1 -- Ideal Rotational Motion Sensor1/RConn2
  Slider-Crank1/RConn1 -- Translational Damper/LConn1 -- Translational Spring/LConn1
  Ideal Torque Sensor1/LConn1 -- Gear Box/LConn1
  Ideal Torque Sensor1/RConn1 -- Ideal Angular Velocity Source/LConn1
  PS-Simulink Converter4/LConn1 -- Ideal Torque Sensor1/RConn2

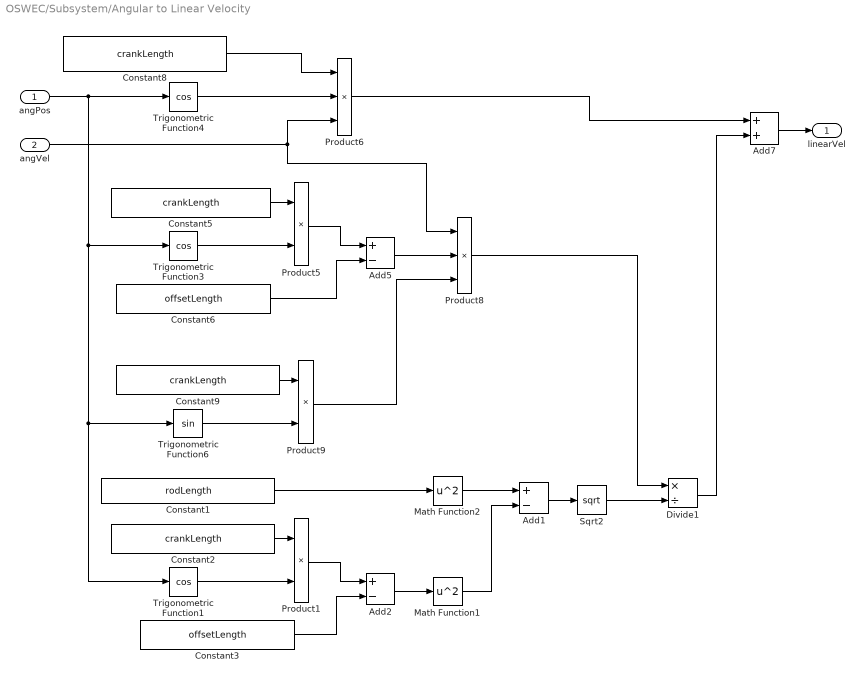
== system OSWEC/Subsystem/Angular to Linear Velocity ==
  angPos : Inport
  angVel : Inport  Port=2
  Add1 : Sum  Inputs=+-
  Add2 : Sum  Inputs=+-
  Add5 : Sum  Inputs=+-
  Add7 : Sum
  Constant1 : Constant  Value=rodLength
  Constant{2,5,8..9} (4 alike) : Constant  Value=crankLength
  Constant3 : Constant  Value=offsetLength
  Constant6 : Constant  Value=offsetLength
  Divide1 : Product  Inputs=*/
  Math Function1 : Math  Operator=square  SignedPower=on
  Math Function2 : Math  Operator=square  SignedPower=on
  Product1 : Product  Inputs=**
  Product5 : Product  Inputs=**
  Product6 : Product  Inputs=***
  Product8 : Product  Inputs=***
  Product9 : Product  Inputs=**
  Sqrt2 : Sqrt
  Trigonometric Function1 : Trigonometry  Operator=cos
  Trigonometric Function3 : Trigonometry  Operator=cos
  Trigonometric Function4 : Trigonometry  Operator=cos
  Trigonometric Function6 : Trigonometry
  linearVel : Outport
  wires:
  Math Function2/1 -> Add1/1
  Divide1/1 -> Add7/2
  Product8/1 -> Divide1/1
  Sqrt2/1 -> Divide1/2
  Math Function1/1 -> Add1/2
  Constant1/1 -> Math Function2/1
  Constant3/1 -> Add2/2
  Product1/1 -> Add2/1
  Trigonometric Function1/1 -> Product1/2
  Constant2/1 -> Product1/1
  Add1/1 -> Sqrt2/1
  Add2/1 -> Math Function1/1
  angPos/1 -> Trigonometric Function4/1, Trigonometric Function3/1, Trigonometric Function6/1, Trigonometric Function1/1
  Product9/1 -> Product8/3
  Add5/1 -> Product8/2
  angVel/1 -> Product6/3, Product8/1
  Trigonometric Function6/1 -> Product9/2
  Constant9/1 -> Product9/1
  Constant6/1 -> Add5/2
  Product5/1 -> Add5/1
  Trigonometric Function3/1 -> Product5/2
  Constant5/1 -> Product5/1
  Product6/1 -> Add7/1
  Constant8/1 -> Product6/1
  Trigonometric Function4/1 -> Product6/2
  Add7/1 -> linearVel/1

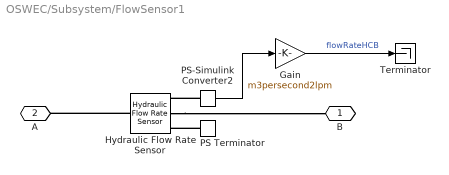
== system OSWEC/Subsystem/FlowSensor1 ==
  Gain : Gain  Gain=m3persecond2lpm
  Hydraulic Flow Rate Sensor : fl_lib/Hydraulic/Hydraulic Sensors/Hydraulic Flow Rate Sensor
  PS Terminator : fl_lib/Physical Signals/Sinks/PS Terminator
  PS-Simulink Converter2 : nesl_utility/PS-Simulink Converter  PhysicalDomain=network_engine_domain  SubClassName=ps_output  LeftPortType=input  RightPortType=output  PseudoPeriodic=off  Frequencies=[]  VectorFormat=inherit  Unit=inherit  AffineConversion=off
  Terminator : Terminator
  B : PMIOPort  Side=Right
  A : PMIOPort  Port=2  Side=Left
  wires:
  PS-Simulink Converter2/1 -> Gain/1
  Gain/1 -> Terminator/1  "flowRateHCB"
  connections:
  Hydraulic Flow Rate Sensor/LConn1 -- A/RConn1
  PS Terminator/LConn1 -- Hydraulic Flow Rate Sensor/RConn3
  PS-Simulink Converter2/LConn1 -- Hydraulic Flow Rate Sensor/RConn1
  Hydraulic Flow Rate Sensor/RConn2 -- B/RConn1

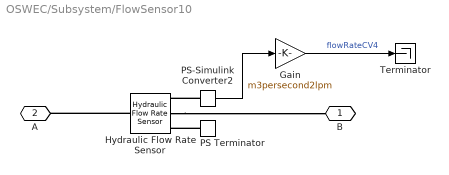
== system OSWEC/Subsystem/FlowSensor10 ==
  Gain : Gain  Gain=m3persecond2lpm
  Hydraulic Flow Rate Sensor : fl_lib/Hydraulic/Hydraulic Sensors/Hydraulic Flow Rate Sensor
  PS Terminator : fl_lib/Physical Signals/Sinks/PS Terminator
  PS-Simulink Converter2 : nesl_utility/PS-Simulink Converter  PhysicalDomain=network_engine_domain  SubClassName=ps_output  LeftPortType=input  RightPortType=output  PseudoPeriodic=off  Frequencies=[]  VectorFormat=inherit  Unit=inherit  AffineConversion=off
  Terminator : Terminator
  B : PMIOPort  Side=Right
  A : PMIOPort  Port=2  Side=Left
  wires:
  PS-Simulink Converter2/1 -> Gain/1
  Gain/1 -> Terminator/1  "flowRateCV4"
  connections:
  Hydraulic Flow Rate Sensor/LConn1 -- A/RConn1
  PS Terminator/LConn1 -- Hydraulic Flow Rate Sensor/RConn3
  PS-Simulink Converter2/LConn1 -- Hydraulic Flow Rate Sensor/RConn1
  Hydraulic Flow Rate Sensor/RConn2 -- B/RConn1

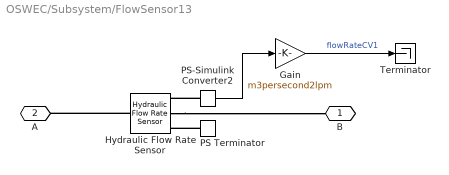
== system OSWEC/Subsystem/FlowSensor13 ==
  Gain : Gain  Gain=m3persecond2lpm
  Hydraulic Flow Rate Sensor : fl_lib/Hydraulic/Hydraulic Sensors/Hydraulic Flow Rate Sensor
  PS Terminator : fl_lib/Physical Signals/Sinks/PS Terminator
  PS-Simulink Converter2 : nesl_utility/PS-Simulink Converter  PhysicalDomain=network_engine_domain  SubClassName=ps_output  LeftPortType=input  RightPortType=output  PseudoPeriodic=off  Frequencies=[]  VectorFormat=inherit  Unit=inherit  AffineConversion=off
  Terminator : Terminator
  B : PMIOPort  Side=Right
  A : PMIOPort  Port=2  Side=Left
  wires:
  PS-Simulink Converter2/1 -> Gain/1
  Gain/1 -> Terminator/1  "flowRateCV1"
  connections:
  Hydraulic Flow Rate Sensor/LConn1 -- A/RConn1
  PS Terminator/LConn1 -- Hydraulic Flow Rate Sensor/RConn3
  PS-Simulink Converter2/LConn1 -- Hydraulic Flow Rate Sensor/RConn1
  Hydraulic Flow Rate Sensor/RConn2 -- B/RConn1

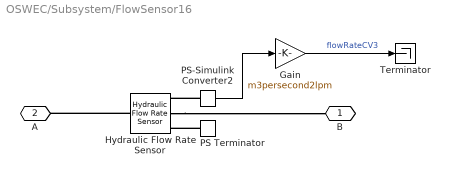
== system OSWEC/Subsystem/FlowSensor16 ==
  Gain : Gain  Gain=m3persecond2lpm
  Hydraulic Flow Rate Sensor : fl_lib/Hydraulic/Hydraulic Sensors/Hydraulic Flow Rate Sensor
  PS Terminator : fl_lib/Physical Signals/Sinks/PS Terminator
  PS-Simulink Converter2 : nesl_utility/PS-Simulink Converter  PhysicalDomain=network_engine_domain  SubClassName=ps_output  LeftPortType=input  RightPortType=output  PseudoPeriodic=off  Frequencies=[]  VectorFormat=inherit  Unit=inherit  AffineConversion=off
  Terminator : Terminator
  B : PMIOPort  Side=Right
  A : PMIOPort  Port=2  Side=Left
  wires:
  PS-Simulink Converter2/1 -> Gain/1
  Gain/1 -> Terminator/1  "flowRateCV3"
  connections:
  Hydraulic Flow Rate Sensor/LConn1 -- A/RConn1
  PS Terminator/LConn1 -- Hydraulic Flow Rate Sensor/RConn3
  PS-Simulink Converter2/LConn1 -- Hydraulic Flow Rate Sensor/RConn1
  Hydraulic Flow Rate Sensor/RConn2 -- B/RConn1

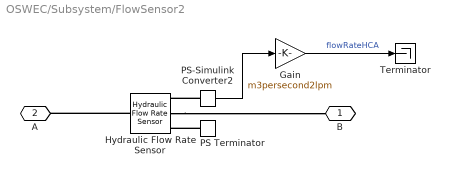
== system OSWEC/Subsystem/FlowSensor2 ==
  Gain : Gain  Gain=m3persecond2lpm
  Hydraulic Flow Rate Sensor : fl_lib/Hydraulic/Hydraulic Sensors/Hydraulic Flow Rate Sensor
  PS Terminator : fl_lib/Physical Signals/Sinks/PS Terminator
  PS-Simulink Converter2 : nesl_utility/PS-Simulink Converter  PhysicalDomain=network_engine_domain  SubClassName=ps_output  LeftPortType=input  RightPortType=output  PseudoPeriodic=off  Frequencies=[]  VectorFormat=inherit  Unit=inherit  AffineConversion=off
  Terminator : Terminator
  B : PMIOPort  Side=Right
  A : PMIOPort  Port=2  Side=Left
  wires:
  PS-Simulink Converter2/1 -> Gain/1
  Gain/1 -> Terminator/1  "flowRateHCA"
  connections:
  Hydraulic Flow Rate Sensor/LConn1 -- A/RConn1
  PS Terminator/LConn1 -- Hydraulic Flow Rate Sensor/RConn3
  PS-Simulink Converter2/LConn1 -- Hydraulic Flow Rate Sensor/RConn1
  Hydraulic Flow Rate Sensor/RConn2 -- B/RConn1

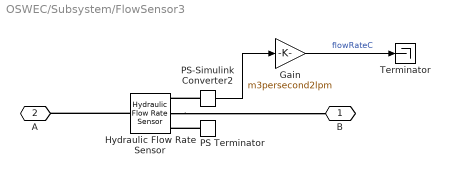
== system OSWEC/Subsystem/FlowSensor3 ==
  Gain : Gain  Gain=m3persecond2lpm
  Hydraulic Flow Rate Sensor : fl_lib/Hydraulic/Hydraulic Sensors/Hydraulic Flow Rate Sensor
  PS Terminator : fl_lib/Physical Signals/Sinks/PS Terminator
  PS-Simulink Converter2 : nesl_utility/PS-Simulink Converter  PhysicalDomain=network_engine_domain  SubClassName=ps_output  LeftPortType=input  RightPortType=output  PseudoPeriodic=off  Frequencies=[]  VectorFormat=inherit  Unit=inherit  AffineConversion=off
  Terminator : Terminator
  B : PMIOPort  Side=Right
  A : PMIOPort  Port=2  Side=Left
  wires:
  PS-Simulink Converter2/1 -> Gain/1
  Gain/1 -> Terminator/1  "flowRateC"
  connections:
  Hydraulic Flow Rate Sensor/LConn1 -- A/RConn1
  PS Terminator/LConn1 -- Hydraulic Flow Rate Sensor/RConn3
  PS-Simulink Converter2/LConn1 -- Hydraulic Flow Rate Sensor/RConn1
  Hydraulic Flow Rate Sensor/RConn2 -- B/RConn1

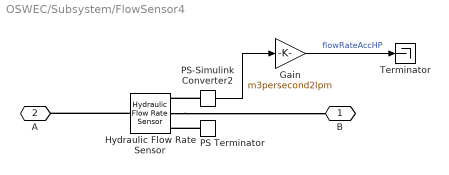
== system OSWEC/Subsystem/FlowSensor4 ==
  Gain : Gain  Gain=m3persecond2lpm
  Hydraulic Flow Rate Sensor : fl_lib/Hydraulic/Hydraulic Sensors/Hydraulic Flow Rate Sensor
  PS Terminator : fl_lib/Physical Signals/Sinks/PS Terminator
  PS-Simulink Converter2 : nesl_utility/PS-Simulink Converter  PhysicalDomain=network_engine_domain  SubClassName=ps_output  LeftPortType=input  RightPortType=output  PseudoPeriodic=off  Frequencies=[]  VectorFormat=inherit  Unit=inherit  AffineConversion=off
  Terminator : Terminator
  B : PMIOPort  Side=Right
  A : PMIOPort  Port=2  Side=Left
  wires:
  PS-Simulink Converter2/1 -> Gain/1
  Gain/1 -> Terminator/1  "flowRateAccHP"
  connections:
  Hydraulic Flow Rate Sensor/LConn1 -- A/RConn1
  PS Terminator/LConn1 -- Hydraulic Flow Rate Sensor/RConn3
  PS-Simulink Converter2/LConn1 -- Hydraulic Flow Rate Sensor/RConn1
  Hydraulic Flow Rate Sensor/RConn2 -- B/RConn1

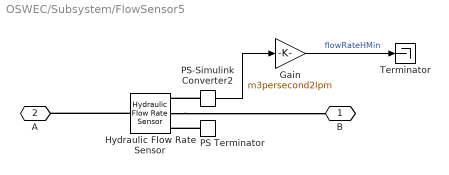
== system OSWEC/Subsystem/FlowSensor5 ==
  Gain : Gain  Gain=m3persecond2lpm
  Hydraulic Flow Rate Sensor : fl_lib/Hydraulic/Hydraulic Sensors/Hydraulic Flow Rate Sensor
  PS Terminator : fl_lib/Physical Signals/Sinks/PS Terminator
  PS-Simulink Converter2 : nesl_utility/PS-Simulink Converter  PhysicalDomain=network_engine_domain  SubClassName=ps_output  LeftPortType=input  RightPortType=output  PseudoPeriodic=off  Frequencies=[]  VectorFormat=inherit  Unit=inherit  AffineConversion=off
  Terminator : Terminator
  B : PMIOPort  Side=Right
  A : PMIOPort  Port=2  Side=Left
  wires:
  PS-Simulink Converter2/1 -> Gain/1
  Gain/1 -> Terminator/1  "flowRateHMin"
  connections:
  Hydraulic Flow Rate Sensor/LConn1 -- A/RConn1
  PS Terminator/LConn1 -- Hydraulic Flow Rate Sensor/RConn3
  PS-Simulink Converter2/LConn1 -- Hydraulic Flow Rate Sensor/RConn1
  Hydraulic Flow Rate Sensor/RConn2 -- B/RConn1

== system OSWEC/Subsystem/FlowSensor6 ==
  Gain : Gain  Gain=m3persecond2lpm
  Hydraulic Flow Rate Sensor : fl_lib/Hydraulic/Hydraulic Sensors/Hydraulic Flow Rate Sensor
  PS Terminator : fl_lib/Physical Signals/Sinks/PS Terminator
  PS-Simulink Converter2 : nesl_utility/PS-Simulink Converter  PhysicalDomain=network_engine_domain  SubClassName=ps_output  LeftPortType=input  RightPortType=output  PseudoPeriodic=off  Frequencies=[]  VectorFormat=inherit  Unit=inherit  AffineConversion=off
  Terminator : Terminator
  B : PMIOPort  Side=Right
  A : PMIOPort  Port=2  Side=Left
  wires:
  PS-Simulink Converter2/1 -> Gain/1
  Gain/1 -> Terminator/1  "flowRateHMout"
  connections:
  Hydraulic Flow Rate Sensor/LConn1 -- A/RConn1
  PS Terminator/LConn1 -- Hydraulic Flow Rate Sensor/RConn3
  PS-Simulink Converter2/LConn1 -- Hydraulic Flow Rate Sensor/RConn1
  Hydraulic Flow Rate Sensor/RConn2 -- B/RConn1

== system OSWEC/Subsystem/FlowSensor7 ==
  Gain : Gain  Gain=m3persecond2lpm
  Hydraulic Flow Rate Sensor : fl_lib/Hydraulic/Hydraulic Sensors/Hydraulic Flow Rate Sensor
  PS Terminator : fl_lib/Physical Signals/Sinks/PS Terminator
  PS-Simulink Converter2 : nesl_utility/PS-Simulink Converter  PhysicalDomain=network_engine_domain  SubClassName=ps_output  LeftPortType=input  RightPortType=output  PseudoPeriodic=off  Frequencies=[]  VectorFormat=inherit  Unit=inherit  AffineConversion=off
  Terminator : Terminator
  B : PMIOPort  Side=Right
  A : PMIOPort  Port=2  Side=Left
  wires:
  PS-Simulink Converter2/1 -> Gain/1
  Gain/1 -> Terminator/1  "flowRateAccLP"
  connections:
  Hydraulic Flow Rate Sensor/LConn1 -- A/RConn1
  PS Terminator/LConn1 -- Hydraulic Flow Rate Sensor/RConn3
  PS-Simulink Converter2/LConn1 -- Hydraulic Flow Rate Sensor/RConn1
  Hydraulic Flow Rate Sensor/RConn2 -- B/RConn1

== system OSWEC/Subsystem/FlowSensor8 ==
  Gain : Gain  Gain=m3persecond2lpm
  Hydraulic Flow Rate Sensor : fl_lib/Hydraulic/Hydraulic Sensors/Hydraulic Flow Rate Sensor
  PS Terminator : fl_lib/Physical Signals/Sinks/PS Terminator
  PS-Simulink Converter2 : nesl_utility/PS-Simulink Converter  PhysicalDomain=network_engine_domain  SubClassName=ps_output  LeftPortType=input  RightPortType=output  PseudoPeriodic=off  Frequencies=[]  VectorFormat=inherit  Unit=inherit  AffineConversion=off
  Terminator : Terminator
  B : PMIOPort  Side=Right
  A : PMIOPort  Port=2  Side=Left
  wires:
  PS-Simulink Converter2/1 -> Gain/1
  Gain/1 -> Terminator/1  "flowRateD"
  connections:
  Hydraulic Flow Rate Sensor/LConn1 -- A/RConn1
  PS Terminator/LConn1 -- Hydraulic Flow Rate Sensor/RConn3
  PS-Simulink Converter2/LConn1 -- Hydraulic Flow Rate Sensor/RConn1
  Hydraulic Flow Rate Sensor/RConn2 -- B/RConn1

== system OSWEC/Subsystem/FlowSensor9 ==
  Gain : Gain  Gain=m3persecond2lpm
  Hydraulic Flow Rate Sensor : fl_lib/Hydraulic/Hydraulic Sensors/Hydraulic Flow Rate Sensor
  PS Terminator : fl_lib/Physical Signals/Sinks/PS Terminator
  PS-Simulink Converter2 : nesl_utility/PS-Simulink Converter  PhysicalDomain=network_engine_domain  SubClassName=ps_output  LeftPortType=input  RightPortType=output  PseudoPeriodic=off  Frequencies=[]  VectorFormat=inherit  Unit=inherit  AffineConversion=off
  Terminator : Terminator
  B : PMIOPort  Side=Right
  A : PMIOPort  Port=2  Side=Left
  wires:
  PS-Simulink Converter2/1 -> Gain/1
  Gain/1 -> Terminator/1  "flowRateCV2"
  connections:
  Hydraulic Flow Rate Sensor/LConn1 -- A/RConn1
  PS Terminator/LConn1 -- Hydraulic Flow Rate Sensor/RConn3
  PS-Simulink Converter2/LConn1 -- Hydraulic Flow Rate Sensor/RConn1
  Hydraulic Flow Rate Sensor/RConn2 -- B/RConn1

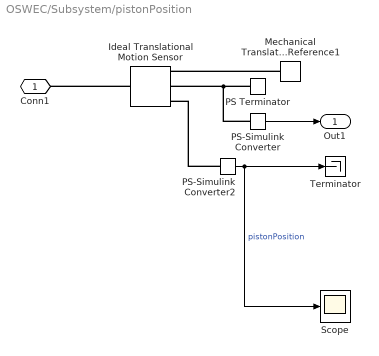
== system OSWEC/Subsystem/pistonPosition ==
  Ideal Translational Motion Sensor : fl_lib/Mechanical/Mechanical Sensors/Ideal Translational Motion Sensor  reference=foundation.enum.MeasurementReference.difference  acceleration_port=false  velocity_port=true  position_port=true  offset=0 m
  Mechanical Translational Reference1 : fl_lib/Mechanical/Translational Elements/Mechanical Translational Reference
  PS Terminator : fl_lib/Physical Signals/Sinks/PS Terminator
  PS-Simulink Converter : nesl_utility/PS-Simulink Converter  PhysicalDomain=network_engine_domain  SubClassName=ps_output  LeftPortType=input  RightPortType=output  PseudoPeriodic=off  Frequencies=[]  VectorFormat=inherit  Unit=inherit  AffineConversion=off
  PS-Simulink Converter2 : nesl_utility/PS-Simulink Converter  PhysicalDomain=network_engine_domain  SubClassName=ps_output  LeftPortType=input  RightPortType=output  PseudoPeriodic=off  Frequencies=[]  VectorFormat=inherit  Unit=inherit  AffineConversion=off
  Scope : Scope
      settings: ActiveDisplayYMinimum=-0.080911717849368445  ActiveDisplayYMaximum=0.6625292550148727  DataLoggingVariableName=ScopeData5
  Terminator : Terminator
  Conn1 : PMIOPort  Side=Left
  Out1 : Outport
  wires:
  PS-Simulink Converter2/1 -> Scope/1, Terminator/1  "pistonPosition"
  PS-Simulink Converter/1 -> Out1/1
  connections:
  Ideal Translational Motion Sensor/LConn1 -- Conn1/RConn1
  PS Terminator/LConn1 -- PS-Simulink Converter/LConn1 -- Ideal Translational Motion Sensor/RConn2
  PS-Simulink Converter2/LConn1 -- Ideal Translational Motion Sensor/RConn3
  Mechanical Translational Reference1/LConn1 -- Ideal Translational Motion Sensor/RConn1

== system OSWEC/Subsystem/pressureSensorA ==
  Gain : Gain  Gain=pa2psi
  Hydraulic Pressure Sensor : fl_lib/Hydraulic/Hydraulic Sensors/Hydraulic Pressure Sensor
  Hydraulic Reference : fl_lib/Hydraulic/Hydraulic Elements/Hydraulic Reference
  PS-Simulink Converter2 : nesl_utility/PS-Simulink Converter  PhysicalDomain=network_engine_domain  SubClassName=ps_output  LeftPortType=input  RightPortType=output  PseudoPeriodic=off  Frequencies=[]  VectorFormat=inherit  Unit=inherit  AffineConversion=off
  Scope : Scope
      settings: ActiveDisplayYMinimum=-108.18611715828341  ActiveDisplayYMaximum=973.67505442455092  DataLoggingVariableName=ScopeData4
  Terminator : Terminator
  Conn1 : PMIOPort  Side=Left
  wires:
  Gain/1 -> Scope/1, Terminator/1  "pressureA"
  PS-Simulink Converter2/1 -> Gain/1
  connections:
  PS-Simulink Converter2/LConn1 -- Hydraulic Pressure Sensor/RConn2
  Hydraulic Reference/LConn1 -- Hydraulic Pressure Sensor/RConn1
  Hydraulic Pressure Sensor/LConn1 -- Conn1/RConn1

== system OSWEC/Subsystem/pressureSensorB ==
  Gain : Gain  Gain=pa2psi
  Hydraulic Pressure Sensor : fl_lib/Hydraulic/Hydraulic Sensors/Hydraulic Pressure Sensor
  Hydraulic Reference : fl_lib/Hydraulic/Hydraulic Elements/Hydraulic Reference
  PS-Simulink Converter2 : nesl_utility/PS-Simulink Converter  PhysicalDomain=network_engine_domain  SubClassName=ps_output  LeftPortType=input  RightPortType=output  PseudoPeriodic=off  Frequencies=[]  VectorFormat=inherit  Unit=inherit  AffineConversion=off
  Scope : Scope
      settings: ActiveDisplayYMinimum=-22.167205478263213  ActiveDisplayYMaximum=1755.5061383660914  DataLoggingVariableName=ScopeData3
  Terminator : Terminator
  Conn1 : PMIOPort  Side=Left
  wires:
  Gain/1 -> Scope/1, Terminator/1  "pressureB"
  PS-Simulink Converter2/1 -> Gain/1
  connections:
  PS-Simulink Converter2/LConn1 -- Hydraulic Pressure Sensor/RConn2
  Hydraulic Reference/LConn1 -- Hydraulic Pressure Sensor/RConn1
  Hydraulic Pressure Sensor/LConn1 -- Conn1/RConn1

== system OSWEC/Subsystem/pressureSensorC ==
  Gain : Gain  Gain=pa2psi
  Hydraulic Pressure Sensor : fl_lib/Hydraulic/Hydraulic Sensors/Hydraulic Pressure Sensor
  Hydraulic Reference : fl_lib/Hydraulic/Hydraulic Elements/Hydraulic Reference
  PS-Simulink Converter2 : nesl_utility/PS-Simulink Converter  PhysicalDomain=network_engine_domain  SubClassName=ps_output  LeftPortType=input  RightPortType=output  PseudoPeriodic=off  Frequencies=[]  VectorFormat=inherit  Unit=inherit  AffineConversion=off
  Terminator : Terminator
  Conn1 : PMIOPort  Side=Left
  wires:
  Gain/1 -> Terminator/1  "pressureC"
  PS-Simulink Converter2/1 -> Gain/1
  connections:
  PS-Simulink Converter2/LConn1 -- Hydraulic Pressure Sensor/RConn2
  Hydraulic Reference/LConn1 -- Hydraulic Pressure Sensor/RConn1
  Hydraulic Pressure Sensor/LConn1 -- Conn1/RConn1

== system OSWEC/Subsystem/pressureSensorC1 ==
  Gain : Gain  Gain=pa2psi
  Hydraulic Pressure Sensor : fl_lib/Hydraulic/Hydraulic Sensors/Hydraulic Pressure Sensor
  Hydraulic Reference : fl_lib/Hydraulic/Hydraulic Elements/Hydraulic Reference
  PS-Simulink Converter2 : nesl_utility/PS-Simulink Converter  PhysicalDomain=network_engine_domain  SubClassName=ps_output  LeftPortType=input  RightPortType=output  PseudoPeriodic=off  Frequencies=[]  VectorFormat=inherit  Unit=inherit  AffineConversion=off
  Scope : Scope
      settings: ActiveDisplayYMinimum=129.86941769572641  ActiveDisplayYMaximum=1541.1272657005441  DataLoggingVariableName=ScopeData6
  Terminator : Terminator
  Conn1 : PMIOPort  Side=Left
  wires:
  Gain/1 -> Scope/1, Terminator/1  "pressureHM"
  PS-Simulink Converter2/1 -> Gain/1
  connections:
  PS-Simulink Converter2/LConn1 -- Hydraulic Pressure Sensor/RConn2
  Hydraulic Reference/LConn1 -- Hydraulic Pressure Sensor/RConn1
  Hydraulic Pressure Sensor/LConn1 -- Conn1/RConn1

== system OSWEC/Subsystem/pressureSensorD ==
  Gain : Gain  Gain=pa2psi
  Hydraulic Pressure Sensor : fl_lib/Hydraulic/Hydraulic Sensors/Hydraulic Pressure Sensor
  Hydraulic Reference : fl_lib/Hydraulic/Hydraulic Elements/Hydraulic Reference
  PS-Simulink Converter2 : nesl_utility/PS-Simulink Converter  PhysicalDomain=network_engine_domain  SubClassName=ps_output  LeftPortType=input  RightPortType=output  PseudoPeriodic=off  Frequencies=[]  VectorFormat=inherit  Unit=inherit  AffineConversion=off
  Scope : Scope
      settings: ActiveDisplayYMinimum=-6.2082719103911472  ActiveDisplayYMaximum=137.72426049135703  DataLoggingVariableName=ScopeData7
  Terminator : Terminator
  Conn1 : PMIOPort  Side=Left
  wires:
  Gain/1 -> Scope/1, Terminator/1  "pressureD"
  PS-Simulink Converter2/1 -> Gain/1
  connections:
  PS-Simulink Converter2/LConn1 -- Hydraulic Pressure Sensor/RConn2
  Hydraulic Reference/LConn1 -- Hydraulic Pressure Sensor/RConn1
  Hydraulic Pressure Sensor/LConn1 -- Conn1/RConn1
